simulink model "gimbal_test_optm_2018_03"  (R2017a)
settings: Solver=ode14x  StartTime=0.0  StopTime=10  FixedStep=0.001  RelTol=1e-3  EnableMultiTasking=on
values from neighbouring files (symbols this model uses):
  m = MAG(:,3:5)    [acc_calibration_t1.m]
  s = tf('s')    [adaptive_control.m]    (also in constraints.m = 1e-19)
undefined symbols (not defined in the file or in its folder): sigbuilder_block, X, Y, Z
libraries: sm_lib x45, nesl_utility x24, simulink x19
(part 1 of 2)
settings Model: Creator=Chaohua Zhao  LastModifiedBy=Chaohua Zhao
settings DataIOCC: LimitDataPoints=on
settings OptimizationCC: LifeSpan=inf
settings DebuggingCC: AllowSymbolicDim=off  SFUnexpectedBacktrackingDiag=warning  SFNoUnconditionalDefaultTransitionDiag=warning  SFExecutionAtInitializationDiag=none
settings ModelReferenceCC: PropagateSignalLabelsOutOfModel=off
settings GRTTargetCC: TargetLangStandard=C89/C90 (ANSI)
settings ConfigComp: CovMetricSettings=dw  CovHtmlReporting=on  CovSaveCumulativeToWorkspaceVar=on  CovSaveSingleToWorkspaceVar=on  CovExternalEMLEnable=off
settings ConfigurationSet: Description=SimMechanics 2G

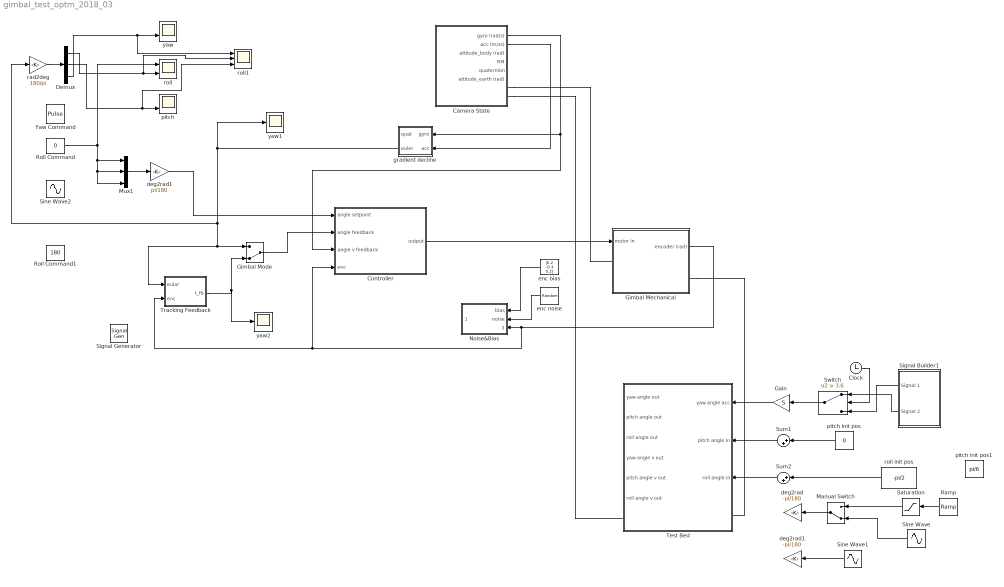
== system gimbal_test_optm_2018_03 ==
  Camera State : Subsystem
  Clock : Clock
  Controller : Subsystem  TreatAsAtomicUnit=on
  Demux : Demux  Outputs=3
  Gain : Gain  Gain=5
  Gimbal Mechanical : Subsystem
  Gimbal Mode : ManualSwitch  CurrentSetting=0
  Manual Switch : ManualSwitch  CurrentSetting=0
  Mux1 : Mux  Inputs=3
  Noise&Bias : Subsystem
  Ramp : simulink/Sources/Ramp  slope=70  start=1  X0=0
  Roll Command : Constant  Value=0
  Roll Command1 : Constant  Value=180
  Saturation : Saturate  UpperLimit=100  LowerLimit=-70
  Signal Generator : SignalGenerator  Units=rad/sec
  Signal Builder1 : Subsystem  Tag=STV Subsys  LoadFcn=sigbuilder_block('load');  StartFcn=sigbuilder_block('start');  StopFcn=sigbuilder_block('stop');  ClipboardFcn=sigbuilder_block('clipboard');  mask(Sigbuilder block){tuvar=[0:10]}
      mask help: Simulink:masks:SigbuilderBlock_MD
      mask init:
      | if ~strcmp(get_param(bdroot(gcbh),'SimulationStatus'),'stopped') tuvar = sigbuilder_block('maskInit'); end
      settings: CopyFcn=sigbuilder_block('copy');  DeleteFcn=sigbuilder_block('delete');  ModelCloseFcn=sigbuilder_block('modelClose');  PreSaveFcn=sigbuilder_block('preSave');  PauseFcn=sigbuilder_block('pause');  ContinueFcn=sigbuilder_block('continue');  NameChangeFcn=sigbuilder_block('namechange');  OpenFcn=sigbuilder_block('open',[6 74.25 1188 459 ]);  CloseFcn=sigbuilder_block('close');
      mask Display: plot(0, 0, 100, 100,[2, 2, 32, 32, 2], [68, 8, 8, 68, 68],[32, 2], [38, 38], [32, 19, 2],[53, 60, 44], [32, 17, 17, 2],[16, 16, 31, 31]);txt = getActiveGroup(gcbh);text(2, 100, txt,'verticalAlignment', 'top');
  Sine Wave : Sin  Amplitude=50  Frequency=2  SampleTime=0
  Sine Wave1 : Sin  Amplitude=60  Frequency=1.7  SampleTime=0
  Sine Wave2 : Sin  Amplitude=270  Frequency=2  SampleTime=0
  Sum1 : Sum  Inputs=|++
  Sum2 : Sum  Inputs=|++
  Switch : Switch  Criteria=u2 > Threshold  Threshold=3.6
  Test Bed : Subsystem
  Tracking Feedback : MATLAB Function  TreatAsAtomicUnit=on
  Yaw Command : DiscretePulseGenerator  PulseType=Time based  Amplitude=90  Period=3  PulseWidth=50
  deg2rad : Gain  Gain=-pi/180
  deg2rad1 : Gain  Gain=-pi/180
  "deg2rad1 " : Gain  Gain=pi/180
  enc bias : Constant  Value=[0.2 -0.3 0.2]
  enc noise : RandomNumber  Variance=0.01  SampleTime=0.001
  gradient decline : Subsystem
  pitch : Scope  NumInputPorts=2
  pitch init pos : Constant  Value=0
  pitch init pos1 : Constant  Value=pi/6
  rad2deg : Gain  Gain=180/pi
  roll : Scope  NumInputPorts=2
  roll init pos : Constant  Value=-pi/2
  roll1 : Scope  NumInputPorts=3
  yaw : Scope  NumInputPorts=2
  yaw1 : Scope
  yaw2 : Scope
  wires:
  pitch init pos/1 -> Sum1/1
  roll init pos/1 -> Sum2/1
  Ramp/1 -> Saturation/1
  Saturation/1 -> Manual Switch/1
  Sine Wave/1 -> Manual Switch/2
  Manual Switch/1 -> deg2rad/1
  Clock/1 -> Switch/2
  Signal Builder1/2(Signal 2) -> Switch/1
  Signal Builder1/1(Signal 1) -> Switch/3
  Sum1/1 -> Test Bed/2(pitch angle in)
  Sum2/1 -> Test Bed/3(roll angle in)
  Sine Wave1/1 -> deg2rad1/1
  Camera State/1(gyro (rad/s)) -> gradient decline/1(gyro), Controller/3(angle v feedback)
  Camera State/2(acc (m/ss)) -> gradient decline/2(acc)
  Gain/1 -> Test Bed/1(yaw angle acc)
  Mux1/1 -> "deg2rad1 "/1
  Controller/1(output) -> Gimbal Mechanical/1(motor in)
  Roll Command/1 -> Mux1/3, Mux1/2, Mux1/1, roll/1
  gradient decline/2("euler ") -> yaw1/1, Gimbal Mode/1, Tracking Feedback/1(eular), rad2deg/1
  Demux/1 -> roll1/2, roll/2
  Demux/2 -> roll1/3, pitch/2
  Demux/3 -> roll1/1, yaw/2
  rad2deg/1 -> Demux/1
  Gimbal Mechanical/1(encoder (rad)) -> Tracking Feedback/2(enc), Controller/4("enc "), Noise&Bias/3(raw enc)
  enc bias/1 -> Noise&Bias/1(bias)
  enc noise/1 -> Noise&Bias/2(noise)
  Tracking Feedback/1(t_fb) -> yaw2/1, Gimbal Mode/2
  Gimbal Mode/1 -> Controller/2(angle feedback)
  "deg2rad1 "/1 -> Controller/1(angle setpoint)
  Switch/1 -> Gain/1
  connections:
  Gimbal Mechanical/RConn1 -- Test Bed/LConn1
  Camera State/RConn1 -- Gimbal Mechanical/LConn1
  Camera State/RConn2 -- Test Bed/RConn1

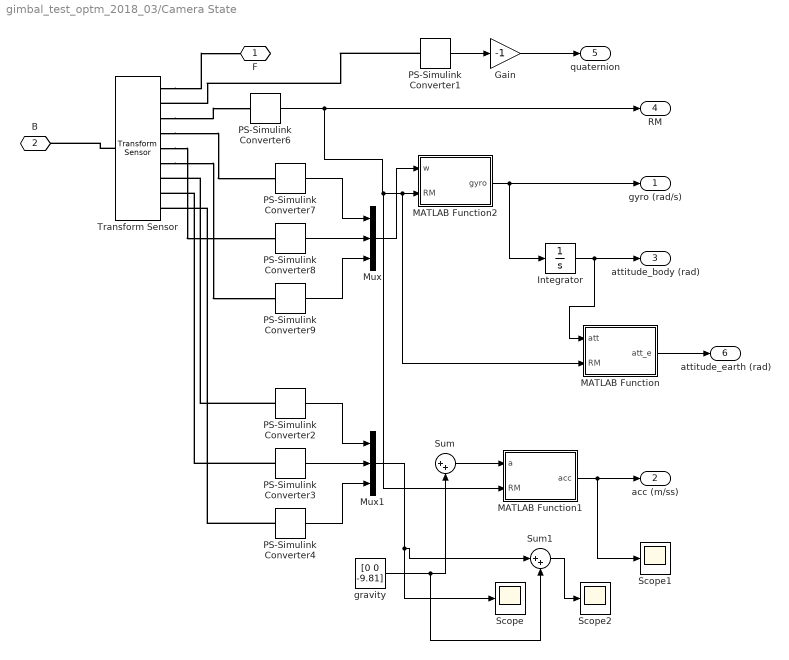
== system gimbal_test_optm_2018_03/Camera State ==
  Gain : Gain  Gain=-1
  Integrator : Integrator
  MATLAB Function : MATLAB Function  TreatAsAtomicUnit=on
  MATLAB Function1 : MATLAB Function  TreatAsAtomicUnit=on
  MATLAB Function2 : MATLAB Function  TreatAsAtomicUnit=on
  Mux : Mux  Inputs=3
  Mux1 : Mux  Inputs=3
  PS-Simulink Converter{1..4,6..9} (8 alike) : nesl_utility/PS-Simulink Converter  PhysicalDomain=network_engine_domain  SubClassName=ps_output  LeftPortType=input  RightPortType=output  PseudoPeriodic=off  Frequencies=[]  Unit=1  AffineConversion=off
  Scope : Scope
  Scope1 : Scope
  Scope2 : Scope
  Sum : Sum  Inputs=|++
  Sum1 : Sum  Inputs=|++
  Transform Sensor : sm_lib/Frames and Transforms/Transform Sensor  MeasurementFrame=World  SenseAngle=off  SenseAxis=off  SenseAngle1=off  SenseAngle2=off  SenseAngle3=off  SenseQ=on  SenseR=on  SenseOmegaX=on  SenseOmegaY=on  SenseOmegaZ=on  SenseOmega1=off  SenseOmega2=off  SenseOmega3=off  SenseQDot=off  SenseRDot=off  SenseAlphaX=off  SenseAlphaY=off  SenseAlphaZ=off  SenseAlpha1=off  SenseAlpha2=off  SenseAlpha3=off  SenseQDDot=off  SenseRDDot=off  SenseX=off  SenseY=off  SenseZ=off  SenseRad=off  SenseAzim=off  SenseDist=off  SenseInc=off  SenseXDot=off  SenseYDot=off  SenseZDot=off  SenseRadDot=off  SenseAzimDot=off  SenseDistDot=off  SenseIncDot=off  SenseXDDot=on  SenseYDDot=on  SenseZDDot=on  SenseRadDDot=off  SenseAzimDDot=off  SenseDistDDot=off  SenseIncDDot=off
  "gravity " : Constant  Value=[0 0 -9.81]
  F : PMIOPort  Port=1  Side=Right
  B : PMIOPort  Port=2  Side=Right
  gyro (rad/s) : Outport
  acc (m/ss) : Outport  Port=2
  attitude_body (rad) : Outport  Port=3
  RM : Outport  Port=4
  "quaternion " : Outport  Port=5
  attitude_earth (rad) : Outport  Port=6
  wires:
  PS-Simulink Converter6/1 -> RM/1, MATLAB Function1/2(RM), MATLAB Function/2(RM), MATLAB Function2/2(RM)
  PS-Simulink Converter7/1 -> Mux/1
  PS-Simulink Converter9/1 -> Mux/3
  MATLAB Function2/1(gyro) -> gyro (rad/s)/1, Integrator/1
  PS-Simulink Converter8/1 -> Mux/2
  Integrator/1 -> MATLAB Function/1(att), attitude_body (rad)/1
  Mux/1 -> MATLAB Function2/1(w)
  PS-Simulink Converter1/1 -> Gain/1
  Gain/1 -> "quaternion "/1
  PS-Simulink Converter3/1 -> Mux1/2
  PS-Simulink Converter4/1 -> Mux1/3
  PS-Simulink Converter2/1 -> Mux1/1
  MATLAB Function1/1(acc) -> Scope1/1, acc (m/ss)/1
  "gravity "/1 -> Sum/2, Sum1/2
  Sum/1 -> MATLAB Function1/1(a)
  Sum1/1 -> Scope2/1
  Mux1/1 -> Sum1/1, Scope/1
  MATLAB Function/1(att_e) -> attitude_earth (rad)/1
  connections:
  Transform Sensor/LConn1 -- B/RConn1
  Transform Sensor/RConn1 -- F/RConn1
  Transform Sensor/RConn6 -- PS-Simulink Converter9/LConn1
  Transform Sensor/RConn5 -- PS-Simulink Converter8/LConn1
  Transform Sensor/RConn4 -- PS-Simulink Converter7/LConn1
  Transform Sensor/RConn3 -- PS-Simulink Converter6/LConn1
  PS-Simulink Converter1/LConn1 -- Transform Sensor/RConn2
  PS-Simulink Converter3/LConn1 -- Transform Sensor/RConn8
  PS-Simulink Converter4/LConn1 -- Transform Sensor/RConn9
  PS-Simulink Converter2/LConn1 -- Transform Sensor/RConn7

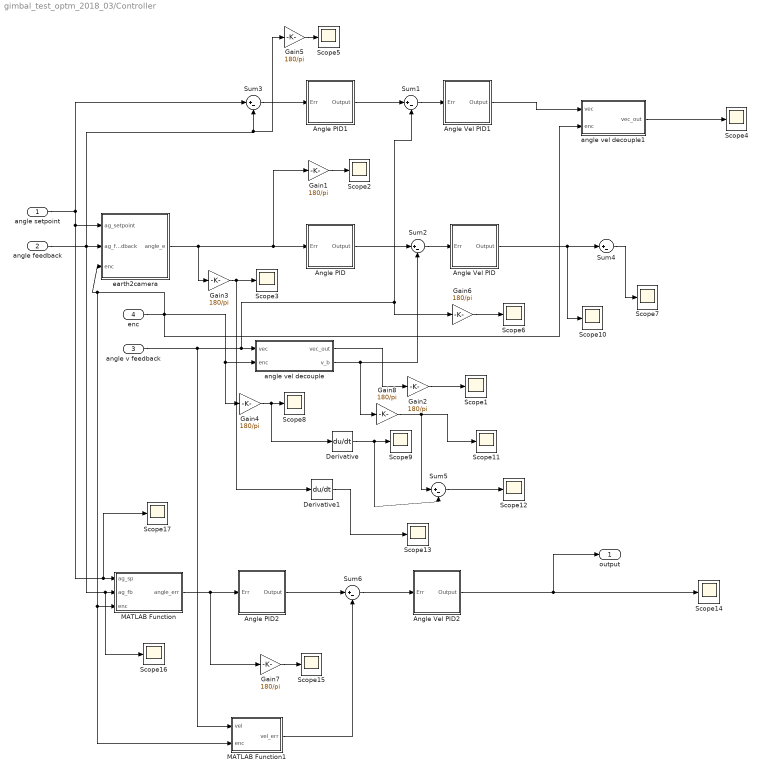
== system gimbal_test_optm_2018_03/Controller ==
  angle setpoint : Inport
  angle feedback : Inport  Port=2
  angle v feedback : Inport  Port=3
  "enc " : Inport  Port=4
  Angle PID : Subsystem
  Angle PID1 : Subsystem
  Angle PID2 : Subsystem
  Angle Vel PID : Subsystem
  Angle Vel PID1 : Subsystem
  Angle Vel PID2 : Subsystem
  Derivative : Derivative
  Derivative1 : Derivative
  Gain{1..8} (8 alike) : Gain  Gain=180/pi
  MATLAB Function : MATLAB Function  TreatAsAtomicUnit=on
  MATLAB Function1 : MATLAB Function  TreatAsAtomicUnit=on
  Scope{1..17} (17 alike) : Scope
  Sum{1..6} (6 alike) : Sum  Inputs=|+-
  angle vel decouple : MATLAB Function  TreatAsAtomicUnit=on
  angle vel decouple1 : MATLAB Function  TreatAsAtomicUnit=on
  earth2camera : MATLAB Function  TreatAsAtomicUnit=on
  output : Outport
  wires:
  angle setpoint/1 -> earth2camera/1(ag_setpoint), Scope17/1, MATLAB Function/1(ag_sp), Sum3/1
  angle feedback/1 -> Scope16/1, MATLAB Function/2(ag_fb), earth2camera/2(ag_feedback), Gain5/1, Sum3/2
  "enc "/1 -> MATLAB Function1/2(enc), MATLAB Function/3(enc), earth2camera/3(enc), angle vel decouple1/2(enc), Gain4/1, angle vel decouple/2(enc)
  angle v feedback/1 -> Sum1/2, Gain6/1, angle vel decouple/1(vec), MATLAB Function1/1(vel)
  angle vel decouple/1(vec_out) -> Gain2/1
  Angle PID1/1(Output) -> Sum1/1
  Sum1/1 -> Angle Vel PID1/1(Err)
  Sum3/1 -> Angle PID1/1(Err)
  Angle Vel PID1/1(Output) -> angle vel decouple1/1(vec)
  Gain1/1 -> Scope2/1
  Gain2/1 -> Scope1/1
  Gain6/1 -> Scope6/1
  Gain5/1 -> Scope5/1
  Sum2/1 -> Angle Vel PID/1(Err)
  Gain4/1 -> Derivative/1, Scope8/1
  Angle Vel PID/1(Output) -> Scope10/1, Sum4/1
  Angle PID/1(Output) -> Sum2/1
  angle vel decouple1/1(vec_out) -> Scope4/1
  Sum4/1 -> Scope7/1
  Gain3/1 -> Scope3/1, Derivative1/1
  earth2camera/1(angle_e) -> Gain3/1, Angle PID/1(Err), Gain1/1
  Derivative/1 -> Sum5/2, Scope9/1
  Sum5/1 -> Scope12/1
  Gain8/1 -> Scope11/1, Sum5/1
  Derivative1/1 -> Scope13/1
  Angle PID2/1(Output) -> Sum6/1
  Sum6/1 -> Angle Vel PID2/1(Err)
  angle vel decouple/2(v_b) -> Gain8/1, Sum2/2
  Angle Vel PID2/1(Output) -> Scope14/1, output/1
  MATLAB Function/1(angle_err) -> Gain7/1, Angle PID2/1(Err)
  Gain7/1 -> Scope15/1
  MATLAB Function1/1(vel_err) -> Sum6/2

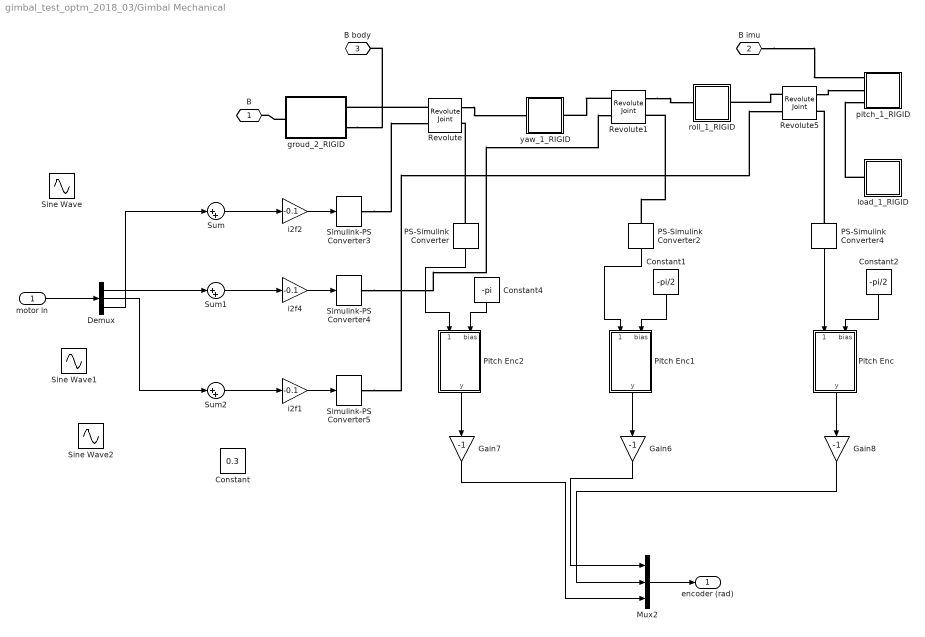
== system gimbal_test_optm_2018_03/Gimbal Mechanical ==
  motor in : Inport
  Constant : Constant  Value=0.3
  Constant1 : Constant  Value=-pi/2
  Constant2 : Constant  Value=-pi/2
  Constant4 : Constant  Value=-pi
  Demux : Demux  Outputs=3
  Gain6 : Gain  Gain=-1
  Gain7 : Gain  Gain=-1
  Gain8 : Gain  Gain=-1
  Mux2 : Mux  Inputs=3
  PS-Simulink Converter : nesl_utility/PS-Simulink Converter  PhysicalDomain=network_engine_domain  SubClassName=ps_output  LeftPortType=input  RightPortType=output  PseudoPeriodic=off  Frequencies=[]  Unit=1  AffineConversion=off
  PS-Simulink Converter2 : nesl_utility/PS-Simulink Converter  PhysicalDomain=network_engine_domain  SubClassName=ps_output  LeftPortType=input  RightPortType=output  PseudoPeriodic=off  Frequencies=[]  Unit=1  AffineConversion=off
  PS-Simulink Converter4 : nesl_utility/PS-Simulink Converter  PhysicalDomain=network_engine_domain  SubClassName=ps_output  LeftPortType=input  RightPortType=output  PseudoPeriodic=off  Frequencies=[]  Unit=1  AffineConversion=off
  Pitch Enc : MATLAB Function  TreatAsAtomicUnit=on
  Pitch Enc1 : MATLAB Function  TreatAsAtomicUnit=on
  Pitch Enc2 : MATLAB Function  TreatAsAtomicUnit=on
  Revolute : sm_lib/Joints/Revolute Joint  SenseConstraintForce=off  SenseConstraintForceX=off  SenseConstraintForceY=off  SenseConstraintForceZ=off  SenseConstraintTorque=off  SenseConstraintTorqueX=off  SenseConstraintTorqueY=off  SenseConstraintTorqueZ=off  SenseTotalForce=off  SenseTotalForceX=off  SenseTotalForceY=off  SenseTotalForceZ=off  SenseTotalTorque=off  SenseTotalTorqueX=off  SenseTotalTorqueY=off  SenseTotalTorqueZ=off  CompositeWrenchDir=FollowerOnBase  CompositeWrenchFrame=BaseFrame  EquilibriumPosition=0  EquilibriumPositionUnits=rad  SpringStiffness=0  SpringStiffnessUnits=m*N/rad  DampingCoefficient=0  DampingCoefficientUnits=m*s*N/rad  TorqueActuationMode=InputTorque  MotionActuationMode=ComputedMotion  SensePosition=on  SenseVelocity=off  SenseAcceleration=off  SenseTorqueForce=off  PositionTargetSpecify=on  PositionTargetPriority=Low  PositionTargetValue=180  PositionTargetValueUnits=deg  VelocityTargetSpecify=off  VelocityTargetPriority=High  VelocityTargetValue=0  VelocityTargetValueUnits=deg/s
  Revolute1 : sm_lib/Joints/Revolute Joint  SenseConstraintForce=off  SenseConstraintForceX=off  SenseConstraintForceY=off  SenseConstraintForceZ=off  SenseConstraintTorque=off  SenseConstraintTorqueX=off  SenseConstraintTorqueY=off  SenseConstraintTorqueZ=off  SenseTotalForce=off  SenseTotalForceX=off  SenseTotalForceY=off  SenseTotalForceZ=off  SenseTotalTorque=off  SenseTotalTorqueX=off  SenseTotalTorqueY=off  SenseTotalTorqueZ=off  CompositeWrenchDir=FollowerOnBase  CompositeWrenchFrame=BaseFrame  EquilibriumPosition=0  EquilibriumPositionUnits=rad  SpringStiffness=0  SpringStiffnessUnits=m*N/rad  DampingCoefficient=0  DampingCoefficientUnits=m*s*N/rad  TorqueActuationMode=InputTorque  MotionActuationMode=ComputedMotion  SensePosition=on  SenseVelocity=off  SenseAcceleration=off  SenseTorqueForce=off  PositionTargetSpecify=on  PositionTargetPriority=Low  PositionTargetValue=90  PositionTargetValueUnits=deg  VelocityTargetSpecify=off  VelocityTargetPriority=High  VelocityTargetValue=0  VelocityTargetValueUnits=deg/s
  Revolute5 : sm_lib/Joints/Revolute Joint  SenseConstraintForce=off  SenseConstraintForceX=off  SenseConstraintForceY=off  SenseConstraintForceZ=off  SenseConstraintTorque=off  SenseConstraintTorqueX=off  SenseConstraintTorqueY=off  SenseConstraintTorqueZ=off  SenseTotalForce=off  SenseTotalForceX=off  SenseTotalForceY=off  SenseTotalForceZ=off  SenseTotalTorque=off  SenseTotalTorqueX=off  SenseTotalTorqueY=off  SenseTotalTorqueZ=off  CompositeWrenchDir=FollowerOnBase  CompositeWrenchFrame=BaseFrame  EquilibriumPosition=0  EquilibriumPositionUnits=rad  SpringStiffness=0  SpringStiffnessUnits=m*N/rad  DampingCoefficient=0  DampingCoefficientUnits=m*s*N/rad  TorqueActuationMode=InputTorque  MotionActuationMode=ComputedMotion  SensePosition=on  SenseVelocity=off  SenseAcceleration=off  SenseTorqueForce=off  PositionTargetSpecify=on  PositionTargetPriority=Low  PositionTargetValue=90  PositionTargetValueUnits=deg  VelocityTargetSpecify=off  VelocityTargetPriority=High  VelocityTargetValue=0  VelocityTargetValueUnits=deg/s
  Simulink-PS Converter3 : nesl_utility/Simulink-PS Converter  PhysicalDomain=network_engine_domain  SubClassName=ps_input  LeftPortType=input  RightPortType=output  PseudoPeriodic=off  Frequencies=[]  NoiseDistribution=none  NoiseParameters=[]  Unit=1  AffineConversion=off  FilteringAndDerivatives=zero  SimscapeFilterOrder=1  InputFilterTimeConstant=0.001  UdotUserProvided=1
  Simulink-PS Converter4 : nesl_utility/Simulink-PS Converter  PhysicalDomain=network_engine_domain  SubClassName=ps_input  LeftPortType=input  RightPortType=output  PseudoPeriodic=off  Frequencies=[]  NoiseDistribution=none  NoiseParameters=[]  Unit=1  AffineConversion=off  FilteringAndDerivatives=zero  SimscapeFilterOrder=1  InputFilterTimeConstant=0.001  UdotUserProvided=1
  Simulink-PS Converter5 : nesl_utility/Simulink-PS Converter  PhysicalDomain=network_engine_domain  SubClassName=ps_input  LeftPortType=input  RightPortType=output  PseudoPeriodic=off  Frequencies=[]  NoiseDistribution=none  NoiseParameters=[]  Unit=1  AffineConversion=off  FilteringAndDerivatives=zero  SimscapeFilterOrder=1  InputFilterTimeConstant=0.001  UdotUserProvided=1
  Sine Wave : Sin  Amplitude=11  Frequency=2  SampleTime=0
  Sine Wave1 : Sin  Amplitude=11  Frequency=2.5  SampleTime=0
  Sine Wave2 : Sin  Amplitude=10  Frequency=2.5  SampleTime=0
  Sum : Sum  Inputs=|++
  Sum1 : Sum  Inputs=|++
  Sum2 : Sum  Inputs=|++
  groud_2_RIGID : Subsystem
  i2f1 : Gain  Gain=-0.1
  i2f2 : Gain  Gain=-0.1
  i2f4 : Gain  Gain=-0.1
  load_1_RIGID : Subsystem
  pitch_1_RIGID : Subsystem
  roll_1_RIGID : Subsystem
  yaw_1_RIGID : Subsystem
  B : PMIOPort  Port=1  Side=Right
  B imu : PMIOPort  Port=2  Side=Left
  B body : PMIOPort  Port=3  Side=Left
  encoder (rad) : Outport
  wires:
  PS-Simulink Converter2/1 -> Pitch Enc1/1(angle)
  Constant1/1 -> Pitch Enc1/2(bias)
  Constant4/1 -> Pitch Enc2/2(bias)
  Constant2/1 -> Pitch Enc/2(bias)
  PS-Simulink Converter/1 -> Pitch Enc2/1(angle)
  PS-Simulink Converter4/1 -> Pitch Enc/1(angle)
  Pitch Enc1/1(y) -> Gain6/1
  Pitch Enc/1(y) -> Gain8/1
  Pitch Enc2/1(y) -> Gain7/1
  Gain7/1 -> Mux2/3
  Gain8/1 -> Mux2/2
  i2f4/1 -> Simulink-PS Converter4/1
  i2f1/1 -> Simulink-PS Converter5/1
  i2f2/1 -> Simulink-PS Converter3/1
  Gain6/1 -> Mux2/1
  ? -> ?
  Mux2/1 -> encoder (rad)/1
  motor in/1 -> Demux/1
  Sum/1 -> i2f2/1
  Demux/3 -> Sum/1
  Sum1/1 -> i2f4/1
  Demux/1 -> Sum1/1
  Sum2/1 -> i2f1/1
  Demux/2 -> Sum2/1
  connections:
  Revolute5/RConn1 -- pitch_1_RIGID/LConn2
  Revolute1/LConn1 -- yaw_1_RIGID/RConn1
  Revolute1/RConn1 -- roll_1_RIGID/LConn1
  Revolute/LConn1 -- groud_2_RIGID/RConn1
  groud_2_RIGID/LConn1 -- B/RConn1
  Revolute/RConn1 -- yaw_1_RIGID/LConn1
  load_1_RIGID/LConn1 -- pitch_1_RIGID/LConn3
  Revolute5/LConn1 -- roll_1_RIGID/RConn1
  Simulink-PS Converter5/RConn1 -- Revolute5/LConn2
  PS-Simulink Converter4/LConn1 -- Revolute5/RConn2
  PS-Simulink Converter/LConn1 -- Revolute/RConn2
  PS-Simulink Converter2/LConn1 -- Revolute1/RConn2
  Simulink-PS Converter3/RConn1 -- Revolute/LConn2
  Simulink-PS Converter4/RConn1 -- Revolute1/LConn2
  B imu/RConn1 -- pitch_1_RIGID/LConn1
  groud_2_RIGID/RConn2 -- B body/RConn1

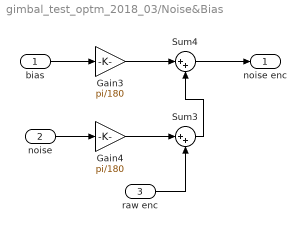
== system gimbal_test_optm_2018_03/Noise&Bias ==
  bias : Inport
  noise : Inport  Port=2
  raw enc : Inport  Port=3
  Gain3 : Gain  Gain=pi/180
  Gain4 : Gain  Gain=pi/180
  Sum3 : Sum  Inputs=|++
  Sum4 : Sum  Inputs=|++
  noise enc : Outport
  wires:
  noise/1 -> Gain4/1
  bias/1 -> Gain3/1
  Gain3/1 -> Sum4/1
  Gain4/1 -> Sum3/1
  raw enc/1 -> Sum3/2
  Sum3/1 -> Sum4/2
  Sum4/1 -> noise enc/1

== system gimbal_test_optm_2018_03/Signal Builder1 ==
  Demux : Demux  Tag=STV Demux  Outputs=2
  FromWs : FromWorkspace  Tag=STV FromWs  VariableName=tuvar  SampleTime=0
      SigBuilderData=|
      | common.afterFinalStr = 'Extrapolate'
      | common.sampleTime = 0
      | dataSet.timeRange = [0 10]
      | dataSet.name = 'Group 1'
      | sbobj.Groups.Name = 'Group 1'
      | sbobj.Groups.Signals(1).Name = 'Signal 1'
      | sbobj.Groups.Signals(1).XData = [0 2.9 3.1 3.2 3.4 10]
      | sbobj.Groups.Signals(1).YData = [0 0 1 1 -0.005 0]
      | sbobj.Groups.Signals(2).Name = 'Signal 2'
      | sbobj.Groups.Signals(2).XData = [0 3.9 4.1 4.2 4.4 10]
      | sbobj.Groups.Signals(2).YData = [0 0 -1 -1 0 0]
  Signal 1 : Outport  Tag=STV Outport
  Signal 2 : Outport  Tag=STV Outport  Port=2
  wires:
  Demux/1 -> Signal 1/1
  FromWs/1 -> Demux/1
  Demux/2 -> Signal 2/1

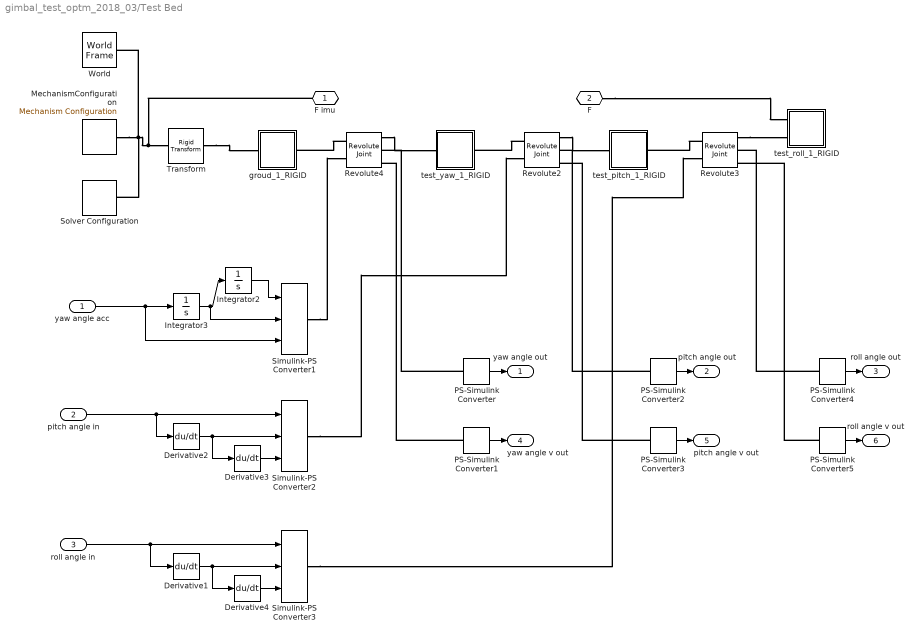
== system gimbal_test_optm_2018_03/Test Bed ==
  yaw angle acc : Inport
  pitch angle in : Inport  Port=2
  roll angle in : Inport  Port=3
  Derivative{1..4} (4 alike) : Derivative
  Integrator2 : Integrator
  Integrator3 : Integrator
  MechanismConfiguration : sm_lib/Utilities/Mechanism Configuration  UniformGravity=Constant  GravityVector=[0 0 -9.81]  GravityUnits=m/s^2  LinearizationDelta=0.001
  PS-Simulink Converter{,1..5} (6 alike) : nesl_utility/PS-Simulink Converter  PhysicalDomain=network_engine_domain  SubClassName=ps_output  LeftPortType=input  RightPortType=output  PseudoPeriodic=off  Frequencies=[]  Unit=1  AffineConversion=off
  Revolute2 : sm_lib/Joints/Revolute Joint  SenseConstraintForce=off  SenseConstraintForceX=off  SenseConstraintForceY=off  SenseConstraintForceZ=off  SenseConstraintTorque=off  SenseConstraintTorqueX=off  SenseConstraintTorqueY=off  SenseConstraintTorqueZ=off  SenseTotalForce=off  SenseTotalForceX=off  SenseTotalForceY=off  SenseTotalForceZ=off  SenseTotalTorque=off  SenseTotalTorqueX=off  SenseTotalTorqueY=off  SenseTotalTorqueZ=off  CompositeWrenchDir=FollowerOnBase  CompositeWrenchFrame=BaseFrame  EquilibriumPosition=0  EquilibriumPositionUnits=rad  SpringStiffness=0  SpringStiffnessUnits=m*N/rad  DampingCoefficient=0  DampingCoefficientUnits=m*s*N/rad  TorqueActuationMode=ComputedTorque  MotionActuationMode=InputMotion  SensePosition=on  SenseVelocity=on  SenseAcceleration=off  SenseTorqueForce=off  PositionTargetSpecify=off  PositionTargetPriority=High  PositionTargetValue=0  PositionTargetValueUnits=deg  VelocityTargetSpecify=off  VelocityTargetPriority=High  VelocityTargetValue=0  VelocityTargetValueUnits=deg/s
  Revolute3 : sm_lib/Joints/Revolute Joint  SenseConstraintForce=off  SenseConstraintForceX=off  SenseConstraintForceY=off  SenseConstraintForceZ=off  SenseConstraintTorque=off  SenseConstraintTorqueX=off  SenseConstraintTorqueY=off  SenseConstraintTorqueZ=off  SenseTotalForce=off  SenseTotalForceX=off  SenseTotalForceY=off  SenseTotalForceZ=off  SenseTotalTorque=off  SenseTotalTorqueX=off  SenseTotalTorqueY=off  SenseTotalTorqueZ=off  CompositeWrenchDir=FollowerOnBase  CompositeWrenchFrame=BaseFrame  EquilibriumPosition=0  EquilibriumPositionUnits=rad  SpringStiffness=0  SpringStiffnessUnits=m*N/rad  DampingCoefficient=0  DampingCoefficientUnits=m*s*N/rad  TorqueActuationMode=ComputedTorque  MotionActuationMode=InputMotion  SensePosition=on  SenseVelocity=on  SenseAcceleration=off  SenseTorqueForce=off  PositionTargetSpecify=on  PositionTargetPriority=Low  PositionTargetValue=70.269058625743583  PositionTargetValueUnits=deg  VelocityTargetSpecify=off  VelocityTargetPriority=High  VelocityTargetValue=0  VelocityTargetValueUnits=deg/s
  Revolute4 : sm_lib/Joints/Revolute Joint  SenseConstraintForce=off  SenseConstraintForceX=off  SenseConstraintForceY=off  SenseConstraintForceZ=off  SenseConstraintTorque=off  SenseConstraintTorqueX=off  SenseConstraintTorqueY=off  SenseConstraintTorqueZ=off  SenseTotalForce=off  SenseTotalForceX=off  SenseTotalForceY=off  SenseTotalForceZ=off  SenseTotalTorque=off  SenseTotalTorqueX=off  SenseTotalTorqueY=off  SenseTotalTorqueZ=off  CompositeWrenchDir=FollowerOnBase  CompositeWrenchFrame=BaseFrame  EquilibriumPosition=0  EquilibriumPositionUnits=rad  SpringStiffness=0  SpringStiffnessUnits=m*N/rad  DampingCoefficient=0  DampingCoefficientUnits=m*s*N/rad  TorqueActuationMode=ComputedTorque  MotionActuationMode=InputMotion  SensePosition=on  SenseVelocity=on  SenseAcceleration=off  SenseTorqueForce=off  PositionTargetSpecify=on  PositionTargetPriority=Low  PositionTargetValue=147.78278879911423  PositionTargetValueUnits=deg  VelocityTargetSpecify=off  VelocityTargetPriority=High  VelocityTargetValue=0  VelocityTargetValueUnits=deg/s
  Simulink-PS Converter1 : nesl_utility/Simulink-PS Converter  PhysicalDomain=network_engine_domain  SubClassName=ps_input  LeftPortType=input  RightPortType=output  PseudoPeriodic=off  Frequencies=[]  NoiseDistribution=none  NoiseParameters=[]  Unit=1  AffineConversion=off  FilteringAndDerivatives=provide  SimscapeFilterOrder=1  InputFilterTimeConstant=0.001  UdotUserProvided=2
  Simulink-PS Converter2 : nesl_utility/Simulink-PS Converter  PhysicalDomain=network_engine_domain  SubClassName=ps_input  LeftPortType=input  RightPortType=output  PseudoPeriodic=off  Frequencies=[]  NoiseDistribution=none  NoiseParameters=[]  Unit=1  AffineConversion=off  FilteringAndDerivatives=provide  SimscapeFilterOrder=1  InputFilterTimeConstant=0.001  UdotUserProvided=2
  Simulink-PS Converter3 : nesl_utility/Simulink-PS Converter  PhysicalDomain=network_engine_domain  SubClassName=ps_input  LeftPortType=input  RightPortType=output  PseudoPeriodic=off  Frequencies=[]  NoiseDistribution=none  NoiseParameters=[]  Unit=1  AffineConversion=off  FilteringAndDerivatives=provide  SimscapeFilterOrder=1  InputFilterTimeConstant=0.001  UdotUserProvided=2
  Solver Configuration : nesl_utility/Solver Configuration  PhysicalDomain=network_engine_domain  SubClassName=solver  LeftPortType=input  RightPortType=generic  Accelerate=off  Tones=[]  Harmonics=[]  SimulateNoise=off  Profile=off  UseLocalSampling=off  EnableSwitchedLinearOptims=on  FrequencyDomain=off  UseCCode=off  RelTol=0.001  AbsTol=1e-06  MinStep=1e-09  ToWorkspace=off  RevertToSquareIcSolve=off  NumHomotopyIterations=100  PhasorMode=off  PhasorModeNumHarmonics=1  OverrideAbsTol=off  DoDC=off  ResidualTolerance=1e-09  UseLocalSolver=off  LocalSolverChoice=NE_BACKWARD_EULER_ADVANCER  LocalSolverSampleTime=0.001  DoFixedCost=off  MaxNonlinIter=3  MaxModeIter=2  LinearAlgebra=Sparse  DelaysMemoryBudget=1024  AutomaticFiltering=on  FilteringTimeConstant=0.001
  Transform : sm_lib/Frames and Transforms/Rigid Transform  TranslationMethod=Cartesian  TranslationStandardOffset=0  TranslationLengthUnit=mm  TranslationStandardAxis=+Z  TranslationCartesianOffset=[3.2381648972062655 30.790535925156188 57.399389346895354]  TranslationROffset=0  TranslationROffsetUnits=m  TranslationZOffset=0  TranslationZOffsetUnits=m  TranslationThetaOffset=0  TranslationThetaOffsetUnits=deg  RotationMethod=ArbitraryAxis  RotationAngleUnits=rad  RotationStandardAxis=+Z  RotationAngle=2.0943951023931913  RotationArbitraryAxis=[0.5773502691896224 0.57735026918963239 0.5773502691896224]  FollAlignAxisA=+X  BaseAlignAxisA=+Y  FollAlignAxisB=+Y  BaseAlignAxisB=+Z  RotationSequenceAxes=FollowerAxes  RotationSequence=XYX  RotationSequenceAngles=[0 0 0]  RotationSequenceAnglesUnits=deg  RotationMatrix=[1 0 0; 0 1 0; 0 0 1]
  World : sm_lib/Frames and Transforms/World Frame
  groud_1_RIGID : Subsystem
  test_pitch_1_RIGID : Subsystem
  test_roll_1_RIGID : Subsystem
  test_yaw_1_RIGID : Subsystem
  "F imu " : PMIOPort  Port=1  Side=Right
  F : PMIOPort  Port=2  Side=Left
  yaw angle out : Outport
  pitch angle out : Outport  Port=2
  roll angle out : Outport  Port=3
  yaw angle v out : Outport  Port=4
  pitch angle v out : Outport  Port=5
  roll angle v out : Outport  Port=6
  wires:
  PS-Simulink Converter1/1 -> yaw angle v out/1
  PS-Simulink Converter3/1 -> pitch angle v out/1
  PS-Simulink Converter/1 -> yaw angle out/1
  PS-Simulink Converter4/1 -> roll angle out/1
  PS-Simulink Converter2/1 -> pitch angle out/1
  PS-Simulink Converter5/1 -> roll angle v out/1
  Derivative2/1 -> Derivative3/1, Simulink-PS Converter2/2
  Derivative3/1 -> Simulink-PS Converter2/3
  Integrator3/1 -> Simulink-PS Converter1/2, Integrator2/1
  Derivative1/1 -> Simulink-PS Converter3/2, Derivative4/1
  Derivative4/1 -> Simulink-PS Converter3/3
  yaw angle acc/1 -> Simulink-PS Converter1/3, Integrator3/1
  roll angle in/1 -> Derivative1/1, Simulink-PS Converter3/1
  pitch angle in/1 -> Derivative2/1, Simulink-PS Converter2/1
  Integrator2/1 -> Simulink-PS Converter1/1
  connections:
  Revolute2/LConn1 -- test_yaw_1_RIGID/RConn1
  Revolute4/LConn1 -- groud_1_RIGID/RConn1
  Revolute3/RConn1 -- test_roll_1_RIGID/LConn2
  Revolute3/LConn1 -- test_pitch_1_RIGID/RConn1
  Revolute4/RConn1 -- test_yaw_1_RIGID/LConn1
  Transform/RConn1 -- groud_1_RIGID/LConn1
  MechanismConfiguration/RConn1 -- Solver Configuration/RConn1 -- World/RConn1 -- "F imu "/RConn1 -- Transform/LConn1
  Revolute2/RConn1 -- test_pitch_1_RIGID/LConn1
  F/RConn1 -- test_roll_1_RIGID/LConn1
  PS-Simulink Converter4/LConn1 -- Revolute3/RConn2
  PS-Simulink Converter1/LConn1 -- Revolute4/RConn3
  PS-Simulink Converter3/LConn1 -- Revolute2/RConn3
  PS-Simulink Converter2/LConn1 -- Revolute2/RConn2
  PS-Simulink Converter5/LConn1 -- Revolute3/RConn3
  Simulink-PS Converter2/RConn1 -- Revolute2/LConn2
  Simulink-PS Converter1/RConn1 -- Revolute4/LConn2
  Simulink-PS Converter3/RConn1 -- Revolute3/LConn2
  PS-Simulink Converter/LConn1 -- Revolute4/RConn2

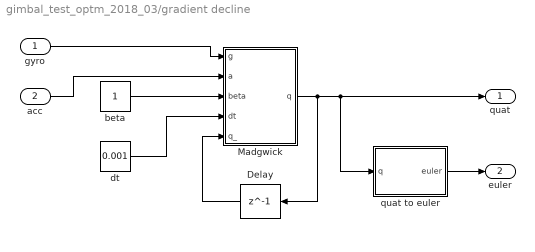
== system gimbal_test_optm_2018_03/gradient decline ==
  gyro : Inport
  acc : Inport  Port=2
  Delay : Delay  DelayLength=1  InitialCondition=[1;0;0;0]
  Madgwick : MATLAB Function  TreatAsAtomicUnit=on
  beta : Constant
  dt : Constant  Value=0.001
  quat to euler : MATLAB Function  TreatAsAtomicUnit=on
  quat : Outport
  "euler " : Outport  Port=2
  wires:
  acc/1 -> Madgwick/2(a)
  gyro/1 -> Madgwick/1(g)
  Madgwick/1(q) -> quat/1, quat to euler/1(q), Delay/1
  Delay/1 -> Madgwick/5(q_)
  beta/1 -> Madgwick/3(beta)
  dt/1 -> Madgwick/4(dt)
  quat to euler/1(euler) -> "euler "/1

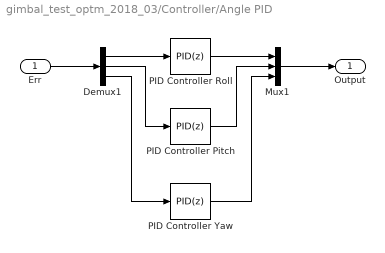
== system gimbal_test_optm_2018_03/Controller/Angle PID ==
  Err : Inport
  Demux1 : Demux  Outputs=3
  Mux1 : Mux  Inputs=3
  PID Controller Pitch : simulink/Continuous/PID Controller  Controller=PID  TimeDomain=Discrete-time  SampleTime=-1  IntegratorMethod=Forward Euler  FilterMethod=Forward Euler  Form=Parallel  UseFilter=on  ControllerParametersSource=internal  P=10  I=0  D=1  N=20  InitialConditionSource=internal  InitialConditionForIntegrator=0  InitialConditionForFilter=0  ExternalReset=none  LimitOutput=on  UpperSaturationLimit=6  LowerSaturationLimit=-6  LinearizeAsGain=on  AntiWindupMode=none  Kb=1  TrackingMode=off  Kt=1  PParamMin=[]  PParamMax=[]  IParamMin=[]  IParamMax=[]  DParamMin=[]  DParamMax=[]  NParamMin=[]  NParamMax=[]  KbParamMin=[]  KbParamMax=[]  KtParamMin=[]  KtParamMax=[]  POutMin=[]  POutMax=[]  IOutMin=[]  IOutMax=[]  DOutMin=[]  DOutMax=[]  NOutMin=[]  NOutMax=[]  KbOutMin=[]  KbOutMax=[]  KtOutMin=[]  KtOutMax=[]  IntegratorOutMin=[]  IntegratorOutMax=[]  FilterOutMin=[]  FilterOutMax=[]  SumOutMin=[]  SumOutMax=[]  SumI1OutMin=[]  SumI1OutMax=[]  SumI2OutMin=[]  SumI2OutMax=[]  SumI3OutMin=[]  SumI3OutMax=[]  SumDOutMin=[]  SumDOutMax=[]  SaturationOutMin=[]  SaturationOutMax=[]  IntegratorContinuousStateAttributes=''  IntegratorStateMustResolveToSignalObject=off  IntegratorRTWStateStorageClass=Auto  FilterContinuousStateAttributes=''  FilterStateMustResolveToSignalObject=off  FilterRTWStateStorageClass=Auto  DifferentiatorICPrevScaledInput=0  DifferentiatorOutMin=[]  DifferentiatorOutMax=[]  InitialConditionSetting=State (most efficient)
  PID Controller Roll : simulink/Continuous/PID Controller  Controller=PID  TimeDomain=Discrete-time  SampleTime=-1  IntegratorMethod=Forward Euler  FilterMethod=Forward Euler  Form=Parallel  UseFilter=on  ControllerParametersSource=internal  P=10  I=0  D=1  N=20  InitialConditionSource=internal  InitialConditionForIntegrator=0  InitialConditionForFilter=0  ExternalReset=none  LimitOutput=on  UpperSaturationLimit=6  LowerSaturationLimit=-6  LinearizeAsGain=on  AntiWindupMode=none  Kb=1  TrackingMode=off  Kt=1  PParamMin=[]  PParamMax=[]  IParamMin=[]  IParamMax=[]  DParamMin=[]  DParamMax=[]  NParamMin=[]  NParamMax=[]  KbParamMin=[]  KbParamMax=[]  KtParamMin=[]  KtParamMax=[]  POutMin=[]  POutMax=[]  IOutMin=[]  IOutMax=[]  DOutMin=[]  DOutMax=[]  NOutMin=[]  NOutMax=[]  KbOutMin=[]  KbOutMax=[]  KtOutMin=[]  KtOutMax=[]  IntegratorOutMin=[]  IntegratorOutMax=[]  FilterOutMin=[]  FilterOutMax=[]  SumOutMin=[]  SumOutMax=[]  SumI1OutMin=[]  SumI1OutMax=[]  SumI2OutMin=[]  SumI2OutMax=[]  SumI3OutMin=[]  SumI3OutMax=[]  SumDOutMin=[]  SumDOutMax=[]  SaturationOutMin=[]  SaturationOutMax=[]  IntegratorContinuousStateAttributes=''  IntegratorStateMustResolveToSignalObject=off  IntegratorRTWStateStorageClass=Auto  FilterContinuousStateAttributes=''  FilterStateMustResolveToSignalObject=off  FilterRTWStateStorageClass=Auto  DifferentiatorICPrevScaledInput=0  DifferentiatorOutMin=[]  DifferentiatorOutMax=[]  InitialConditionSetting=State (most efficient)
  PID Controller Yaw : simulink/Continuous/PID Controller  Controller=PID  TimeDomain=Discrete-time  SampleTime=-1  IntegratorMethod=Forward Euler  FilterMethod=Forward Euler  Form=Parallel  UseFilter=on  ControllerParametersSource=internal  P=10  I=0  D=1  N=1  InitialConditionSource=internal  InitialConditionForIntegrator=0  InitialConditionForFilter=0  ExternalReset=none  LimitOutput=on  UpperSaturationLimit=6  LowerSaturationLimit=-6  LinearizeAsGain=on  AntiWindupMode=none  Kb=1  TrackingMode=off  Kt=1  PParamMin=[]  PParamMax=[]  IParamMin=[]  IParamMax=[]  DParamMin=[]  DParamMax=[]  NParamMin=[]  NParamMax=[]  KbParamMin=[]  KbParamMax=[]  KtParamMin=[]  KtParamMax=[]  POutMin=[]  POutMax=[]  IOutMin=[]  IOutMax=[]  DOutMin=[]  DOutMax=[]  NOutMin=[]  NOutMax=[]  KbOutMin=[]  KbOutMax=[]  KtOutMin=[]  KtOutMax=[]  IntegratorOutMin=[]  IntegratorOutMax=[]  FilterOutMin=[]  FilterOutMax=[]  SumOutMin=[]  SumOutMax=[]  SumI1OutMin=[]  SumI1OutMax=[]  SumI2OutMin=[]  SumI2OutMax=[]  SumI3OutMin=[]  SumI3OutMax=[]  SumDOutMin=[]  SumDOutMax=[]  SaturationOutMin=[]  SaturationOutMax=[]  IntegratorContinuousStateAttributes=''  IntegratorStateMustResolveToSignalObject=off  IntegratorRTWStateStorageClass=Auto  FilterContinuousStateAttributes=''  FilterStateMustResolveToSignalObject=off  FilterRTWStateStorageClass=Auto  DifferentiatorICPrevScaledInput=0  DifferentiatorOutMin=[]  DifferentiatorOutMax=[]  InitialConditionSetting=State (most efficient)
  Output : Outport
  wires:
  Err/1 -> Demux1/1
  Demux1/3 -> PID Controller Yaw/1
  PID Controller Roll/1 -> Mux1/1
  PID Controller Pitch/1 -> Mux1/2
  PID Controller Yaw/1 -> Mux1/3
  Demux1/2 -> PID Controller Pitch/1
  Mux1/1 -> Output/1
  Demux1/1 -> PID Controller Roll/1

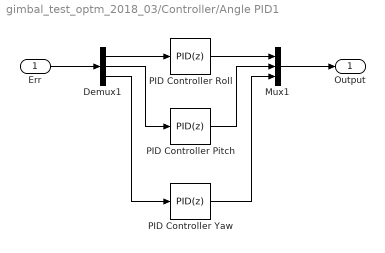
== system gimbal_test_optm_2018_03/Controller/Angle PID1 ==
  Err : Inport
  Demux1 : Demux  Outputs=3
  Mux1 : Mux  Inputs=3
  PID Controller Pitch : simulink/Continuous/PID Controller  Controller=PID  TimeDomain=Discrete-time  SampleTime=-1  IntegratorMethod=Forward Euler  FilterMethod=Forward Euler  Form=Parallel  UseFilter=on  ControllerParametersSource=internal  P=10  I=0  D=1  N=20  InitialConditionSource=internal  InitialConditionForIntegrator=0  InitialConditionForFilter=0  ExternalReset=none  LimitOutput=on  UpperSaturationLimit=6  LowerSaturationLimit=-6  LinearizeAsGain=on  AntiWindupMode=none  Kb=1  TrackingMode=off  Kt=1  PParamMin=[]  PParamMax=[]  IParamMin=[]  IParamMax=[]  DParamMin=[]  DParamMax=[]  NParamMin=[]  NParamMax=[]  KbParamMin=[]  KbParamMax=[]  KtParamMin=[]  KtParamMax=[]  POutMin=[]  POutMax=[]  IOutMin=[]  IOutMax=[]  DOutMin=[]  DOutMax=[]  NOutMin=[]  NOutMax=[]  KbOutMin=[]  KbOutMax=[]  KtOutMin=[]  KtOutMax=[]  IntegratorOutMin=[]  IntegratorOutMax=[]  FilterOutMin=[]  FilterOutMax=[]  SumOutMin=[]  SumOutMax=[]  SumI1OutMin=[]  SumI1OutMax=[]  SumI2OutMin=[]  SumI2OutMax=[]  SumI3OutMin=[]  SumI3OutMax=[]  SumDOutMin=[]  SumDOutMax=[]  SaturationOutMin=[]  SaturationOutMax=[]  IntegratorContinuousStateAttributes=''  IntegratorStateMustResolveToSignalObject=off  IntegratorRTWStateStorageClass=Auto  FilterContinuousStateAttributes=''  FilterStateMustResolveToSignalObject=off  FilterRTWStateStorageClass=Auto  DifferentiatorICPrevScaledInput=0  DifferentiatorOutMin=[]  DifferentiatorOutMax=[]  InitialConditionSetting=State (most efficient)
  PID Controller Roll : simulink/Continuous/PID Controller  Controller=PID  TimeDomain=Discrete-time  SampleTime=-1  IntegratorMethod=Forward Euler  FilterMethod=Forward Euler  Form=Parallel  UseFilter=on  ControllerParametersSource=internal  P=10  I=0  D=1  N=20  InitialConditionSource=internal  InitialConditionForIntegrator=0  InitialConditionForFilter=0  ExternalReset=none  LimitOutput=on  UpperSaturationLimit=6  LowerSaturationLimit=-6  LinearizeAsGain=on  AntiWindupMode=none  Kb=1  TrackingMode=off  Kt=1  PParamMin=[]  PParamMax=[]  IParamMin=[]  IParamMax=[]  DParamMin=[]  DParamMax=[]  NParamMin=[]  NParamMax=[]  KbParamMin=[]  KbParamMax=[]  KtParamMin=[]  KtParamMax=[]  POutMin=[]  POutMax=[]  IOutMin=[]  IOutMax=[]  DOutMin=[]  DOutMax=[]  NOutMin=[]  NOutMax=[]  KbOutMin=[]  KbOutMax=[]  KtOutMin=[]  KtOutMax=[]  IntegratorOutMin=[]  IntegratorOutMax=[]  FilterOutMin=[]  FilterOutMax=[]  SumOutMin=[]  SumOutMax=[]  SumI1OutMin=[]  SumI1OutMax=[]  SumI2OutMin=[]  SumI2OutMax=[]  SumI3OutMin=[]  SumI3OutMax=[]  SumDOutMin=[]  SumDOutMax=[]  SaturationOutMin=[]  SaturationOutMax=[]  IntegratorContinuousStateAttributes=''  IntegratorStateMustResolveToSignalObject=off  IntegratorRTWStateStorageClass=Auto  FilterContinuousStateAttributes=''  FilterStateMustResolveToSignalObject=off  FilterRTWStateStorageClass=Auto  DifferentiatorICPrevScaledInput=0  DifferentiatorOutMin=[]  DifferentiatorOutMax=[]  InitialConditionSetting=State (most efficient)
  PID Controller Yaw : simulink/Continuous/PID Controller  Controller=PID  TimeDomain=Discrete-time  SampleTime=-1  IntegratorMethod=Forward Euler  FilterMethod=Forward Euler  Form=Parallel  UseFilter=on  ControllerParametersSource=internal  P=10  I=0  D=1  N=1  InitialConditionSource=internal  InitialConditionForIntegrator=0  InitialConditionForFilter=0  ExternalReset=none  LimitOutput=on  UpperSaturationLimit=6  LowerSaturationLimit=-6  LinearizeAsGain=on  AntiWindupMode=none  Kb=1  TrackingMode=off  Kt=1  PParamMin=[]  PParamMax=[]  IParamMin=[]  IParamMax=[]  DParamMin=[]  DParamMax=[]  NParamMin=[]  NParamMax=[]  KbParamMin=[]  KbParamMax=[]  KtParamMin=[]  KtParamMax=[]  POutMin=[]  POutMax=[]  IOutMin=[]  IOutMax=[]  DOutMin=[]  DOutMax=[]  NOutMin=[]  NOutMax=[]  KbOutMin=[]  KbOutMax=[]  KtOutMin=[]  KtOutMax=[]  IntegratorOutMin=[]  IntegratorOutMax=[]  FilterOutMin=[]  FilterOutMax=[]  SumOutMin=[]  SumOutMax=[]  SumI1OutMin=[]  SumI1OutMax=[]  SumI2OutMin=[]  SumI2OutMax=[]  SumI3OutMin=[]  SumI3OutMax=[]  SumDOutMin=[]  SumDOutMax=[]  SaturationOutMin=[]  SaturationOutMax=[]  IntegratorContinuousStateAttributes=''  IntegratorStateMustResolveToSignalObject=off  IntegratorRTWStateStorageClass=Auto  FilterContinuousStateAttributes=''  FilterStateMustResolveToSignalObject=off  FilterRTWStateStorageClass=Auto  DifferentiatorICPrevScaledInput=0  DifferentiatorOutMin=[]  DifferentiatorOutMax=[]  InitialConditionSetting=State (most efficient)
  Output : Outport
  wires:
  Demux1/1 -> PID Controller Roll/1
  Mux1/1 -> Output/1
  Demux1/2 -> PID Controller Pitch/1
  PID Controller Yaw/1 -> Mux1/3
  PID Controller Pitch/1 -> Mux1/2
  PID Controller Roll/1 -> Mux1/1
  Demux1/3 -> PID Controller Yaw/1
  Err/1 -> Demux1/1

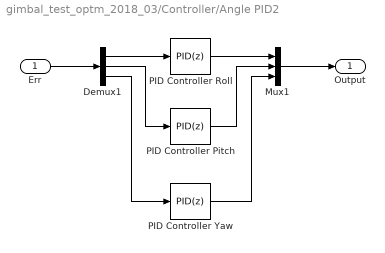
== system gimbal_test_optm_2018_03/Controller/Angle PID2 ==
  Err : Inport
  Demux1 : Demux  Outputs=3
  Mux1 : Mux  Inputs=3
  PID Controller Pitch : simulink/Continuous/PID Controller  Controller=PID  TimeDomain=Discrete-time  SampleTime=-1  IntegratorMethod=Forward Euler  FilterMethod=Forward Euler  Form=Parallel  UseFilter=on  ControllerParametersSource=internal  P=10  I=0  D=1  N=20  InitialConditionSource=internal  InitialConditionForIntegrator=0  InitialConditionForFilter=0  ExternalReset=none  LimitOutput=on  UpperSaturationLimit=6  LowerSaturationLimit=-6  LinearizeAsGain=on  AntiWindupMode=none  Kb=1  TrackingMode=off  Kt=1  PParamMin=[]  PParamMax=[]  IParamMin=[]  IParamMax=[]  DParamMin=[]  DParamMax=[]  NParamMin=[]  NParamMax=[]  KbParamMin=[]  KbParamMax=[]  KtParamMin=[]  KtParamMax=[]  POutMin=[]  POutMax=[]  IOutMin=[]  IOutMax=[]  DOutMin=[]  DOutMax=[]  NOutMin=[]  NOutMax=[]  KbOutMin=[]  KbOutMax=[]  KtOutMin=[]  KtOutMax=[]  IntegratorOutMin=[]  IntegratorOutMax=[]  FilterOutMin=[]  FilterOutMax=[]  SumOutMin=[]  SumOutMax=[]  SumI1OutMin=[]  SumI1OutMax=[]  SumI2OutMin=[]  SumI2OutMax=[]  SumI3OutMin=[]  SumI3OutMax=[]  SumDOutMin=[]  SumDOutMax=[]  SaturationOutMin=[]  SaturationOutMax=[]  IntegratorContinuousStateAttributes=''  IntegratorStateMustResolveToSignalObject=off  IntegratorRTWStateStorageClass=Auto  FilterContinuousStateAttributes=''  FilterStateMustResolveToSignalObject=off  FilterRTWStateStorageClass=Auto  DifferentiatorICPrevScaledInput=0  DifferentiatorOutMin=[]  DifferentiatorOutMax=[]  InitialConditionSetting=State (most efficient)
  PID Controller Roll : simulink/Continuous/PID Controller  Controller=PID  TimeDomain=Discrete-time  SampleTime=-1  IntegratorMethod=Forward Euler  FilterMethod=Forward Euler  Form=Parallel  UseFilter=on  ControllerParametersSource=internal  P=10  I=0  D=1  N=20  InitialConditionSource=internal  InitialConditionForIntegrator=0  InitialConditionForFilter=0  ExternalReset=none  LimitOutput=on  UpperSaturationLimit=6  LowerSaturationLimit=-6  LinearizeAsGain=on  AntiWindupMode=none  Kb=1  TrackingMode=off  Kt=1  PParamMin=[]  PParamMax=[]  IParamMin=[]  IParamMax=[]  DParamMin=[]  DParamMax=[]  NParamMin=[]  NParamMax=[]  KbParamMin=[]  KbParamMax=[]  KtParamMin=[]  KtParamMax=[]  POutMin=[]  POutMax=[]  IOutMin=[]  IOutMax=[]  DOutMin=[]  DOutMax=[]  NOutMin=[]  NOutMax=[]  KbOutMin=[]  KbOutMax=[]  KtOutMin=[]  KtOutMax=[]  IntegratorOutMin=[]  IntegratorOutMax=[]  FilterOutMin=[]  FilterOutMax=[]  SumOutMin=[]  SumOutMax=[]  SumI1OutMin=[]  SumI1OutMax=[]  SumI2OutMin=[]  SumI2OutMax=[]  SumI3OutMin=[]  SumI3OutMax=[]  SumDOutMin=[]  SumDOutMax=[]  SaturationOutMin=[]  SaturationOutMax=[]  IntegratorContinuousStateAttributes=''  IntegratorStateMustResolveToSignalObject=off  IntegratorRTWStateStorageClass=Auto  FilterContinuousStateAttributes=''  FilterStateMustResolveToSignalObject=off  FilterRTWStateStorageClass=Auto  DifferentiatorICPrevScaledInput=0  DifferentiatorOutMin=[]  DifferentiatorOutMax=[]  InitialConditionSetting=State (most efficient)
  PID Controller Yaw : simulink/Continuous/PID Controller  Controller=PID  TimeDomain=Discrete-time  SampleTime=-1  IntegratorMethod=Forward Euler  FilterMethod=Forward Euler  Form=Parallel  UseFilter=on  ControllerParametersSource=internal  P=10  I=0  D=1  N=1  InitialConditionSource=internal  InitialConditionForIntegrator=0  InitialConditionForFilter=0  ExternalReset=none  LimitOutput=on  UpperSaturationLimit=6  LowerSaturationLimit=-6  LinearizeAsGain=on  AntiWindupMode=none  Kb=1  TrackingMode=off  Kt=1  PParamMin=[]  PParamMax=[]  IParamMin=[]  IParamMax=[]  DParamMin=[]  DParamMax=[]  NParamMin=[]  NParamMax=[]  KbParamMin=[]  KbParamMax=[]  KtParamMin=[]  KtParamMax=[]  POutMin=[]  POutMax=[]  IOutMin=[]  IOutMax=[]  DOutMin=[]  DOutMax=[]  NOutMin=[]  NOutMax=[]  KbOutMin=[]  KbOutMax=[]  KtOutMin=[]  KtOutMax=[]  IntegratorOutMin=[]  IntegratorOutMax=[]  FilterOutMin=[]  FilterOutMax=[]  SumOutMin=[]  SumOutMax=[]  SumI1OutMin=[]  SumI1OutMax=[]  SumI2OutMin=[]  SumI2OutMax=[]  SumI3OutMin=[]  SumI3OutMax=[]  SumDOutMin=[]  SumDOutMax=[]  SaturationOutMin=[]  SaturationOutMax=[]  IntegratorContinuousStateAttributes=''  IntegratorStateMustResolveToSignalObject=off  IntegratorRTWStateStorageClass=Auto  FilterContinuousStateAttributes=''  FilterStateMustResolveToSignalObject=off  FilterRTWStateStorageClass=Auto  DifferentiatorICPrevScaledInput=0  DifferentiatorOutMin=[]  DifferentiatorOutMax=[]  InitialConditionSetting=State (most efficient)
  Output : Outport
  wires:
  Demux1/1 -> PID Controller Roll/1
  Mux1/1 -> Output/1
  Demux1/2 -> PID Controller Pitch/1
  PID Controller Yaw/1 -> Mux1/3
  PID Controller Pitch/1 -> Mux1/2
  PID Controller Roll/1 -> Mux1/1
  Demux1/3 -> PID Controller Yaw/1
  Err/1 -> Demux1/1

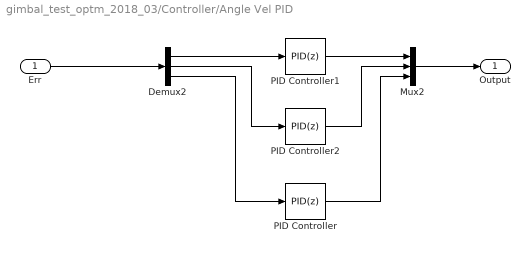
== system gimbal_test_optm_2018_03/Controller/Angle Vel PID ==
  Err : Inport
  Demux2 : Demux  Outputs=3
  Mux2 : Mux  Inputs=3
  PID Controller : simulink/Continuous/PID Controller  Controller=PID  TimeDomain=Discrete-time  SampleTime=-1  IntegratorMethod=Forward Euler  FilterMethod=Forward Euler  Form=Parallel  UseFilter=on  ControllerParametersSource=internal  P=50  I=2  D=0.5  N=1  InitialConditionSource=internal  InitialConditionForIntegrator=0  InitialConditionForFilter=0  ExternalReset=none  LimitOutput=on  UpperSaturationLimit=10  LowerSaturationLimit=-10  LinearizeAsGain=on  AntiWindupMode=none  Kb=1  TrackingMode=off  Kt=1  PParamMin=[]  PParamMax=[]  IParamMin=[]  IParamMax=[]  DParamMin=[]  DParamMax=[]  NParamMin=[]  NParamMax=[]  KbParamMin=[]  KbParamMax=[]  KtParamMin=[]  KtParamMax=[]  POutMin=[]  POutMax=[]  IOutMin=[]  IOutMax=[]  DOutMin=[]  DOutMax=[]  NOutMin=[]  NOutMax=[]  KbOutMin=[]  KbOutMax=[]  KtOutMin=[]  KtOutMax=[]  IntegratorOutMin=[]  IntegratorOutMax=[]  FilterOutMin=[]  FilterOutMax=[]  SumOutMin=[]  SumOutMax=[]  SumI1OutMin=[]  SumI1OutMax=[]  SumI2OutMin=[]  SumI2OutMax=[]  SumI3OutMin=[]  SumI3OutMax=[]  SumDOutMin=[]  SumDOutMax=[]  SaturationOutMin=[]  SaturationOutMax=[]  IntegratorContinuousStateAttributes=''  IntegratorStateMustResolveToSignalObject=off  IntegratorRTWStateStorageClass=Auto  FilterContinuousStateAttributes=''  FilterStateMustResolveToSignalObject=off  FilterRTWStateStorageClass=Auto  DifferentiatorICPrevScaledInput=0  DifferentiatorOutMin=[]  DifferentiatorOutMax=[]  InitialConditionSetting=State (most efficient)
  PID Controller1 : simulink/Continuous/PID Controller  Controller=PID  TimeDomain=Discrete-time  SampleTime=-1  IntegratorMethod=Forward Euler  FilterMethod=Forward Euler  Form=Parallel  UseFilter=on  ControllerParametersSource=internal  P=50  I=0.1  D=0.5  N=20  InitialConditionSource=internal  InitialConditionForIntegrator=0  InitialConditionForFilter=0  ExternalReset=none  LimitOutput=on  UpperSaturationLimit=10  LowerSaturationLimit=-10  LinearizeAsGain=on  AntiWindupMode=none  Kb=1  TrackingMode=off  Kt=1  PParamMin=[]  PParamMax=[]  IParamMin=[]  IParamMax=[]  DParamMin=[]  DParamMax=[]  NParamMin=[]  NParamMax=[]  KbParamMin=[]  KbParamMax=[]  KtParamMin=[]  KtParamMax=[]  POutMin=[]  POutMax=[]  IOutMin=[]  IOutMax=[]  DOutMin=[]  DOutMax=[]  NOutMin=[]  NOutMax=[]  KbOutMin=[]  KbOutMax=[]  KtOutMin=[]  KtOutMax=[]  IntegratorOutMin=[]  IntegratorOutMax=[]  FilterOutMin=[]  FilterOutMax=[]  SumOutMin=[]  SumOutMax=[]  SumI1OutMin=[]  SumI1OutMax=[]  SumI2OutMin=[]  SumI2OutMax=[]  SumI3OutMin=[]  SumI3OutMax=[]  SumDOutMin=[]  SumDOutMax=[]  SaturationOutMin=[]  SaturationOutMax=[]  IntegratorContinuousStateAttributes=''  IntegratorStateMustResolveToSignalObject=off  IntegratorRTWStateStorageClass=Auto  FilterContinuousStateAttributes=''  FilterStateMustResolveToSignalObject=off  FilterRTWStateStorageClass=Auto  DifferentiatorICPrevScaledInput=0  DifferentiatorOutMin=[]  DifferentiatorOutMax=[]  InitialConditionSetting=State (most efficient)
  PID Controller2 : simulink/Continuous/PID Controller  Controller=PID  TimeDomain=Discrete-time  SampleTime=-1  IntegratorMethod=Forward Euler  FilterMethod=Forward Euler  Form=Parallel  UseFilter=on  ControllerParametersSource=internal  P=50  I=0.4  D=0.5  N=20  InitialConditionSource=internal  InitialConditionForIntegrator=0  InitialConditionForFilter=0  ExternalReset=none  LimitOutput=on  UpperSaturationLimit=10  LowerSaturationLimit=-10  LinearizeAsGain=on  AntiWindupMode=none  Kb=1  TrackingMode=off  Kt=1  PParamMin=[]  PParamMax=[]  IParamMin=[]  IParamMax=[]  DParamMin=[]  DParamMax=[]  NParamMin=[]  NParamMax=[]  KbParamMin=[]  KbParamMax=[]  KtParamMin=[]  KtParamMax=[]  POutMin=[]  POutMax=[]  IOutMin=[]  IOutMax=[]  DOutMin=[]  DOutMax=[]  NOutMin=[]  NOutMax=[]  KbOutMin=[]  KbOutMax=[]  KtOutMin=[]  KtOutMax=[]  IntegratorOutMin=[]  IntegratorOutMax=[]  FilterOutMin=[]  FilterOutMax=[]  SumOutMin=[]  SumOutMax=[]  SumI1OutMin=[]  SumI1OutMax=[]  SumI2OutMin=[]  SumI2OutMax=[]  SumI3OutMin=[]  SumI3OutMax=[]  SumDOutMin=[]  SumDOutMax=[]  SaturationOutMin=[]  SaturationOutMax=[]  IntegratorContinuousStateAttributes=''  IntegratorStateMustResolveToSignalObject=off  IntegratorRTWStateStorageClass=Auto  FilterContinuousStateAttributes=''  FilterStateMustResolveToSignalObject=off  FilterRTWStateStorageClass=Auto  DifferentiatorICPrevScaledInput=0  DifferentiatorOutMin=[]  DifferentiatorOutMax=[]  InitialConditionSetting=State (most efficient)
  Output : Outport
  wires:
  Err/1 -> Demux2/1
  Demux2/3 -> PID Controller/1
  Demux2/1 -> PID Controller1/1
  Mux2/1 -> Output/1
  Demux2/2 -> PID Controller2/1
  PID Controller/1 -> Mux2/3
  PID Controller1/1 -> Mux2/1
  PID Controller2/1 -> Mux2/2
